simulink model "gyroPendulum"  (R2018a)
settings: Solver=FixedStepDiscrete  StartTime=0.0  StopTime=inf  FixedStep=timeStep  RelTol=1e-3
values from neighbouring files (symbols this model uses):
  alphaCoefficientsTable = [0.135955504695 0.137071048508 0.137987859192 0.138554072268 0.138582246682 0.137829429264 0.135972150233 0.132577620353 0.127076345916 0.118749819988 0.106761570128 0.0902777777548 ... (122412 elements, 10201x12)]    [cachedAlphaCoefficientsTable.mat]    (also in setup.m = [alphaCoefficientsTable; K1(1, :), K1(2, :)])
  alphaCompareTable = [-171.7 -171.7 -171.7 -171.7 -171.7 -171.7 -171.7 -171.7 -171.7 -171.7 -171.7 -171.7 ... (51005 elements, 10201x5)]    [cachedAlphaCompareTable.mat]    (also in setup.m = [alphaCompareTable; index1 - alphaRegion, index1 + alphaRegi)
  coefficientsTensor = zeros(nLinearizations / nWorkers, nLinearizations, nLinearizations, nLinearizations, 12)    [alphaParallel.m]    (also in coefficientsTensor.mat = [0.0662688248156 0.0648277946669 0.0634135109587 0.062021453)
  K1 = [K1(1, :) K1(2, :)]    [alphaParallel.m]    (also in setup.m = lqr(Aw1, Bw1, diag([1, 1, 3, 1, 1, 1]), diag([6, 6])))
  K2 = lqr(Aw2, Bw2, diag([15, 1, 1, 5]), diag([15]))    [setup.m]
  K3 = lqr(Aw3, Bw3, diag([1, 1, 1, 1]), diag([1]))    [setup.m]
  modelParameters = rmfield(modelParameters, 'alph2')    [alphaParallel.m]    (also in setup.m)
  nLinearizations = 8    [alphaParallel.m]    (also in nLinearizations.mat = 32; setup.m = 100)
  shiftedVariables = [shiftedVariables; wholeVariables(:, 1) + abs(min(wholeVariables(:, 1), [], 2))]    [alphaParallel.m]    (also in shiftedVariables.mat = [0 0 0 0])
  trajectory = [0.204039137261 -0.389047482528 0.184950739835 -0.34807965922 0.208093560422 -0.397377880713 0.182464301801 -0.343183800683 0.212362955443 -0.406162696705 0.180157605825 -0.338633761035 ... (832 elements, 4x208)]    [trajectory.mat]
  trajectoryTimeStep = 0.005    [setup.m]
  trajectoryToWalk = [0.20348839193 -0.387921068139 0.185314050902 -0.348794213842 0.206937106898 -0.395034683488 0.18313781068 -0.34450971149 0.210555704125 -0.402555806913 0.181086396317 -0.340463307968 ... (484 elements, 4x121)]    [trajectoryToWalk.mat]
  trajectoryWalk = [0.250192072849 -0.608547594051 0.394694165643 -0.613804432575 0.251033796696 -0.60716129389 0.397031433715 -0.614641196656 0.251771384595 -0.605603254171 0.399919372114 -0.616088285913 ... (1104 elements, 4x276)]    [trajectoryWalk.mat]
  variablesDeltas = [variablesDeltas; abs(variablesRanges(2:end, 1) - variablesRanges(2:end, 2)) / nLinearizations]    [alphaParallel.m]    (also in variablesDeltas.mat = [16.875 5.625 5.625 5.625])
  variablesShift = [variablesShift; abs(min(wholeVariables, [], 2))]    [alphaParallel.m]    (also in variablesShift.mat = [270 90 90 90])
undefined symbols (not defined in the file or in its folder): DiscIntNeverNeededParam
libraries: simulink x15, dspindex x12, simulink_extras x5
settings Model: EnablePacing=on  PacingRate=2  Creator=Oleg  LastModifiedBy=sorok

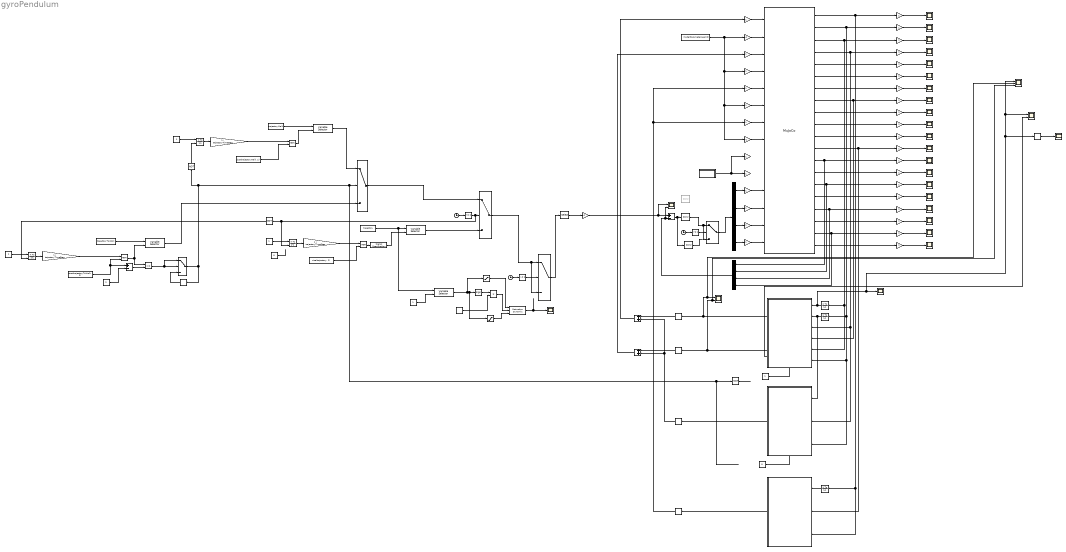
== system gyroPendulum ==
  Add : Sum
  Add1 : Sum
  Clock : Clock
  Clock1 : Clock
  Clock2 : Clock
  Compare To Constant : simulink/Logic and Bit Operations/Compare To Constant  relop=>=  const=2  OutDataTypeStr=boolean
  Compare To Constant1 : simulink/Logic and Bit Operations/Compare To Constant  relop=>=  const=2  OutDataTypeStr=boolean
  Compare To Constant2 : simulink/Logic and Bit Operations/Compare To Constant  relop=>=  const=1  OutDataTypeStr=boolean
  Constant : Constant  Value=modelParameters.gamD
  Constant1 : Constant  Value=size(trajectory, 2)
  Constant10 : Constant  Value=2
  Constant11 : Constant
  Constant12 : Constant  Value=0
  Constant13 : Constant  Value=0
  Constant14 : Constant
  Constant2 : Constant  SampleTime=trajectoryTimeStep
  Constant3 : Constant  Value=trajectory
  Constant4 : Constant  Value=size(trajectoryWalk, 2)
  Constant5 : Constant  SampleTime=trajectoryTimeStep
  Constant6 : Constant  Value=trajectoryWalk
  Constant7 : Constant  Value=size(trajectoryToWalk, 2)
  Constant8 : Constant  SampleTime=trajectoryTimeStep
  Constant9 : Constant  Value=trajectoryToWalk
  Demux : Demux
  Discrete-Time Integrator : DiscreteIntegrator  ExternalReset=level  SampleTime=-1  ICPrevOutput=DiscIntNeverNeededParam  ICPrevScaledInput=DiscIntNeverNeededParam
  Discrete-Time Integrator1 : DiscreteIntegrator  SampleTime=-1  ICPrevOutput=DiscIntNeverNeededParam  ICPrevScaledInput=DiscIntNeverNeededParam
  Discrete-Time Integrator2 : DiscreteIntegrator  SampleTime=-1  ICPrevOutput=DiscIntNeverNeededParam  ICPrevScaledInput=DiscIntNeverNeededParam
  Discrete-Time Integrator3 : DiscreteIntegrator  SampleTime=-1  ICPrevOutput=DiscIntNeverNeededParam  ICPrevScaledInput=DiscIntNeverNeededParam
  Discrete-Time Integrator4 : DiscreteIntegrator  ExternalReset=level  SampleTime=-1  ICPrevOutput=DiscIntNeverNeededParam  ICPrevScaledInput=DiscIntNeverNeededParam
  Discrete-Time Integrator5 : DiscreteIntegrator  ExternalReset=level  SampleTime=-1  ICPrevOutput=DiscIntNeverNeededParam  ICPrevScaledInput=DiscIntNeverNeededParam
  Disturbances : Subsystem
  Equal : RelationalOperator  OutDataTypeStr=boolean  RndMeth=Simplest
  Gain : Gain  Gain=1 / trajectoryTimeStep
  Gain1 : Gain  Gain=1 / trajectoryTimeStep
  Gain2 : Gain  Gain=1 / trajectoryTimeStep
  Gain3 : Gain  Gain=-1
  Memory{,1..4} (5 alike) : Memory
  Minus : Sum  Inputs=+-
  Minus1 : Sum  Inputs=+-
  Multiply : Product
  Mux1 : Mux
  NOT : Logic  Operator=NOT  IconShape=distinctive  AllPortsSameDT=off  OutDataTypeStr=boolean
  NOT1 : Logic  Operator=NOT  IconShape=distinctive  AllPortsSameDT=off  OutDataTypeStr=boolean
  NOT2 : Logic  Operator=NOT  IconShape=distinctive  AllPortsSameDT=off  OutDataTypeStr=boolean
  PID Controller : simulink/Continuous/PID Controller  Controller=PD  TimeDomain=Discrete-time  SampleTime=-1  IntegratorMethod=Forward Euler  FilterMethod=Forward Euler  Form=Parallel  UseFilter=on  ControllerParametersSource=internal  P=350  I=1  D=350  N=100  InitialConditionSource=internal  InitialConditionForIntegrator=0  InitialConditionForFilter=0  ExternalReset=none  LimitOutput=off  UpperSaturationLimit=inf  LowerSaturationLimit=-inf  LinearizeAsGain=on  AntiWindupMode=none  Kb=1  TrackingMode=off  Kt=1  PParamMin=[]  PParamMax=[]  IParamMin=[]  IParamMax=[]  DParamMin=[]  DParamMax=[]  NParamMin=[]  NParamMax=[]  KbParamMin=[]  KbParamMax=[]  KtParamMin=[]  KtParamMax=[]  POutMin=[]  POutMax=[]  IOutMin=[]  IOutMax=[]  DOutMin=[]  DOutMax=[]  NOutMin=[]  NOutMax=[]  KbOutMin=[]  KbOutMax=[]  KtOutMin=[]  KtOutMax=[]  IntegratorOutMin=[]  IntegratorOutMax=[]  FilterOutMin=[]  FilterOutMax=[]  SumOutMin=[]  SumOutMax=[]  SumI1OutMin=[]  SumI1OutMax=[]  SumI2OutMin=[]  SumI2OutMax=[]  SumI3OutMin=[]  SumI3OutMax=[]  SumDOutMin=[]  SumDOutMax=[]  SaturationOutMin=[]  SaturationOutMax=[]  IntegratorContinuousStateAttributes=''  IntegratorStateMustResolveToSignalObject=off  IntegratorRTWStateStorageClass=Auto  FilterContinuousStateAttributes=''  FilterStateMustResolveToSignalObject=off  FilterRTWStateStorageClass=Auto  DifferentiatorICPrevScaledInput=0  DifferentiatorOutMin=[]  DifferentiatorOutMax=[]  FilterDiffOutCoefMin=[]  FilterDiffOutCoefMax=[]  SumDenOutMin=[]  SumDenOutMax=[]  SumNumOutMin=[]  SumNumOutMax=[]  ReciprocalOutMin=[]  ReciprocalOutMax=[]  DivideOutMin=[]  DivideOutMax=[]  TunerSelectOption=Transfer Function Based (PID Tuner App)
  PID Controller1 : simulink/Continuous/PID Controller  Commented=on  Controller=PD  TimeDomain=Discrete-time  SampleTime=-1  IntegratorMethod=Forward Euler  FilterMethod=Forward Euler  Form=Parallel  UseFilter=on  ControllerParametersSource=internal  P=300  I=1  D=300  N=100  InitialConditionSource=internal  InitialConditionForIntegrator=0  InitialConditionForFilter=0  ExternalReset=none  LimitOutput=off  UpperSaturationLimit=inf  LowerSaturationLimit=-inf  LinearizeAsGain=on  AntiWindupMode=none  Kb=1  TrackingMode=off  Kt=1  PParamMin=[]  PParamMax=[]  IParamMin=[]  IParamMax=[]  DParamMin=[]  DParamMax=[]  NParamMin=[]  NParamMax=[]  KbParamMin=[]  KbParamMax=[]  KtParamMin=[]  KtParamMax=[]  POutMin=[]  POutMax=[]  IOutMin=[]  IOutMax=[]  DOutMin=[]  DOutMax=[]  NOutMin=[]  NOutMax=[]  KbOutMin=[]  KbOutMax=[]  KtOutMin=[]  KtOutMax=[]  IntegratorOutMin=[]  IntegratorOutMax=[]  FilterOutMin=[]  FilterOutMax=[]  SumOutMin=[]  SumOutMax=[]  SumI1OutMin=[]  SumI1OutMax=[]  SumI2OutMin=[]  SumI2OutMax=[]  SumI3OutMin=[]  SumI3OutMax=[]  SumDOutMin=[]  SumDOutMax=[]  SaturationOutMin=[]  SaturationOutMax=[]  IntegratorContinuousStateAttributes=''  IntegratorStateMustResolveToSignalObject=off  IntegratorRTWStateStorageClass=Auto  FilterContinuousStateAttributes=''  FilterStateMustResolveToSignalObject=off  FilterRTWStateStorageClass=Auto  DifferentiatorICPrevScaledInput=0  DifferentiatorOutMin=[]  DifferentiatorOutMax=[]  FilterDiffOutCoefMin=[]  FilterDiffOutCoefMax=[]  SumDenOutMin=[]  SumDenOutMax=[]  SumNumOutMin=[]  SumNumOutMax=[]  ReciprocalOutMin=[]  ReciprocalOutMax=[]  DivideOutMin=[]  DivideOutMax=[]  TunerSelectOption=Transfer Function Based (PID Tuner App)
  PID Controller2 : simulink/Continuous/PID Controller  Controller=PD  TimeDomain=Discrete-time  SampleTime=-1  IntegratorMethod=Forward Euler  FilterMethod=Forward Euler  Form=Parallel  UseFilter=on  ControllerParametersSource=internal  P=200  I=1  D=200  N=100  InitialConditionSource=internal  InitialConditionForIntegrator=0  InitialConditionForFilter=0  ExternalReset=none  LimitOutput=off  UpperSaturationLimit=inf  LowerSaturationLimit=-inf  LinearizeAsGain=on  AntiWindupMode=none  Kb=1  TrackingMode=off  Kt=1  PParamMin=[]  PParamMax=[]  IParamMin=[]  IParamMax=[]  DParamMin=[]  DParamMax=[]  NParamMin=[]  NParamMax=[]  KbParamMin=[]  KbParamMax=[]  KtParamMin=[]  KtParamMax=[]  POutMin=[]  POutMax=[]  IOutMin=[]  IOutMax=[]  DOutMin=[]  DOutMax=[]  NOutMin=[]  NOutMax=[]  KbOutMin=[]  KbOutMax=[]  KtOutMin=[]  KtOutMax=[]  IntegratorOutMin=[]  IntegratorOutMax=[]  FilterOutMin=[]  FilterOutMax=[]  SumOutMin=[]  SumOutMax=[]  SumI1OutMin=[]  SumI1OutMax=[]  SumI2OutMin=[]  SumI2OutMax=[]  SumI3OutMin=[]  SumI3OutMax=[]  SumDOutMin=[]  SumDOutMax=[]  SaturationOutMin=[]  SaturationOutMax=[]  IntegratorContinuousStateAttributes=''  IntegratorStateMustResolveToSignalObject=off  IntegratorRTWStateStorageClass=Auto  FilterContinuousStateAttributes=''  FilterStateMustResolveToSignalObject=off  FilterRTWStateStorageClass=Auto  DifferentiatorICPrevScaledInput=0  DifferentiatorOutMin=[]  DifferentiatorOutMax=[]  FilterDiffOutCoefMin=[]  FilterDiffOutCoefMax=[]  SumDenOutMin=[]  SumDenOutMax=[]  SumNumOutMin=[]  SumNumOutMax=[]  ReciprocalOutMin=[]  ReciprocalOutMax=[]  DivideOutMin=[]  DivideOutMax=[]  TunerSelectOption=Transfer Function Based (PID Tuner App)
  Pitch controller (3 dimensions) : Subsystem
  Pitch-yaw controller (7 dimensions) : Subsystem
  Radians to Degrees : simulink_extras/Transformations/Radians to Degrees
  Ramp : simulink/Sources/Ramp  slope=0.2  start=0  InitialOutput=0
  Rem : Math  Operator=rem  SaturateOnIntegerOverflow=on
  Rem1 : Math  Operator=rem  SaturateOnIntegerOverflow=on
  Rem2 : Math  Operator=rem  SaturateOnIntegerOverflow=on
  Roll controller (3 dimensions) : Subsystem
  S-Function : S-Function  FunctionName=MuJoCo  SFunctionDeploymentMode=off  EnableBusSupport=off
  Saturation : Saturate  UpperLimit=inf  LowerLimit=0
  Saturation Dynamic : simulink/Discontinuities/Saturation Dynamic  OutMin=[]  OutMax=[]  OutDataTypeStr=Inherit: Same as second input  OutDataType=fixdt(1, 16)  OutScaling=2^-10  DoSatur=off
  Saturation1 : Saturate  UpperLimit=0  LowerLimit=-inf
  Scope{,1..5,7..21,24,26} (23 alike) : Scope
  Scope22 : Scope  NumInputPorts=3
  Scope23 : Scope  NumInputPorts=2
  Scope25 : Scope  NumInputPorts=2
  Scope6 : Scope  NumInputPorts=2
  Selector1 : Selector  InputPortWidth=4  IndexOptions=Index vector (dialog)  Indices=[3 4 1 2]  OutputSizes=1
  Sign : Signum
  Signal Specification : SignalSpecification  Dimensions=1
  Switch{,1..4} (5 alike) : Switch  Criteria=u2 > Threshold
  Variable Selector{,1..3} (4 alike) : dspindex/Variable Selector  NumInputs=1  rowsOrCols=Columns  IdxMode=Variable  Elements=[1 3]  ZerOneIdxMode=One-based  errmode=Clip Index  FillMode=on  FillValues=0
  gyro1_act : Gain
  gyro1_act_pos : Gain
  gyro1_act_vel : Gain
  gyro1_m : Gain  Gain=-1
  gyro1_m_pos : Gain
  gyro1_m_vel : Gain
  gyro2_act : Gain
  gyro2_act_pos : Gain
  gyro2_act_vel : Gain
  gyro2_m : Gain
  gyro2_m_pos : Gain
  gyro2_m_vel : Gain
  gyro3_act : Gain
  gyro3_act_pos : Gain
  gyro3_m : Gain
  gyro4_act : Gain
  gyro4_m : Gain  Gain=-1
  ls_act : Gain
  ls_pos : Gain
  ls_vel : Gain
  lt_act : Gain
  lt_pos : Gain
  lt_vel : Gain
  rod_act1 : Gain
  rod_act2 : Gain
  rod_x_ang : Gain
  rod_y_ang : Gain
  rod_z_ang : Gain
  rs_act : Gain
  rs_pos : Gain
  rs_vel : Gain
  rt_act : Gain
  rt_pos : Gain
  rt_vel : Gain
  wires:
  rod_x_ang/1 -> Scope/1
  gyro1_act_pos/1 -> Scope2/1
  rod_y_ang/1 -> Scope1/1
  gyro1_act_vel/1 -> Scope3/1
  gyro1_m_pos/1 -> Scope4/1
  gyro1_m_vel/1 -> Scope5/1
  Constant/1 -> gyro4_m/1, gyro3_m/1, gyro2_m/1, gyro1_m/1
  Pitch-yaw controller (7 dimensions)/1(alph1D) -> Scope22/2, Scope6/1, Memory1/1
  Memory1/1 -> Add/1
  gyro1_m/1 -> S-Function/2
  gyro2_act/1 -> S-Function/3
  gyro2_m/1 -> S-Function/4
  gyro2_m_vel/1 -> Scope11/1
  gyro2_m_pos/1 -> Scope10/1
  gyro2_act_vel/1 -> Scope9/1
  gyro2_act_pos/1 -> Scope8/1
  rod_z_ang/1 -> Scope12/1
  Pitch-yaw controller (7 dimensions)/2(alph2D) -> Scope22/3, Scope6/2, Memory2/1
  gyro1_act/1 -> S-Function/1
  Memory2/1 -> Add1/1
  Disturbances/1(Out) -> rod_act1/1, rod_act2/1
  Constant3/1 -> Variable Selector3/1, Variable Selector/1
  Variable Selector/1 -> Switch/3
  Discrete-Time Integrator/1 -> Gain/1
  Constant1/1 -> Rem/2
  Rem/1 -> Signal Specification/1
  Clock/1 -> Compare To Constant/1
  gyro3_m/1 -> S-Function/6
  gyro4_m/1 -> S-Function/8
  gyro3_act/1 -> S-Function/5
  gyro4_act/1 -> S-Function/7
  gyro3_act_pos/1 -> Scope7/1
  Memory3/1 -> gyro3_act/1, gyro4_act/1
  Compare To Constant/1 -> Discrete-Time Integrator/2, NOT/1, Switch/2
  Constant2/1 -> Discrete-Time Integrator/1
  Switch/1 -> Switch3/3, Switch3/1
  S-Function/1 -> Discrete-Time Integrator3/1, Roll controller (3 dimensions)/3(sigmD), rod_x_ang/1
  S-Function/2 -> Discrete-Time Integrator2/1, Pitch controller (3 dimensions)/3(thetD), Pitch-yaw controller (7 dimensions)/6(thetD), rod_y_ang/1
  S-Function/3 -> Discrete-Time Integrator1/1, Pitch-yaw controller (7 dimensions)/5(psihD), rod_z_ang/1
  S-Function/4 -> Pitch-yaw controller (7 dimensions)/3(alph1), Pitch controller (3 dimensions)/2(alph1), gyro1_act_pos/1
  S-Function/5 -> gyro1_act_vel/1
  S-Function/6 -> gyro1_m_pos/1
  S-Function/7 -> gyro1_m_vel/1
  S-Function/8 -> Pitch-yaw controller (7 dimensions)/4(alph2), gyro2_act_pos/1
  S-Function/9 -> gyro2_act_vel/1
  S-Function/10 -> gyro2_m_pos/1
  S-Function/11 -> gyro2_m_vel/1
  S-Function/12 -> gyro3_act_pos/1, Roll controller (3 dimensions)/2(alph3)
  Gain/1 -> Rem/1
  Discrete-Time Integrator1/1 -> Pitch-yaw controller (7 dimensions)/1(psih), Radians to Degrees/1, Scope23/1, Scope22/1, Scope21/1
  Discrete-Time Integrator2/1 -> Pitch-yaw controller (7 dimensions)/2(thet), Pitch controller (3 dimensions)/1(thet)
  Discrete-Time Integrator3/1 -> Roll controller (3 dimensions)/1(sigm)
  S-Function/14 -> lt_vel/1
  S-Function/13 -> Mux1/1, lt_pos/1
  S-Function/15 -> Mux1/2, ls_pos/1
  S-Function/16 -> ls_vel/1
  S-Function/17 -> Mux1/3, rt_pos/1
  S-Function/18 -> rt_vel/1
  S-Function/19 -> Mux1/4, rs_pos/1
  S-Function/20 -> rs_vel/1
  lt_pos/1 -> Scope13/1
  lt_vel/1 -> Scope14/1
  ls_pos/1 -> Scope15/1
  ls_vel/1 -> Scope16/1
  rt_pos/1 -> Scope17/1
  rt_vel/1 -> Scope18/1
  rs_pos/1 -> Scope19/1
  rs_vel/1 -> Scope20/1
  Demux/1 -> lt_act/1
  Demux/2 -> ls_act/1
  Demux/3 -> rt_act/1
  Demux/4 -> rs_act/1
  Minus/1 -> PID Controller2/1, PID Controller/1
  Mux1/1 -> Scope25/2, Minus/2
  Gain1/1 -> Rem1/1
  Constant5/1 -> Discrete-Time Integrator4/1
  Rem1/1 -> Variable Selector1/2
  Constant4/1 -> Rem1/2
  Discrete-Time Integrator4/1 -> Gain1/1
  Variable Selector1/1 -> Switch1/1
  Constant6/1 -> Variable Selector1/1
  NOT/1 -> Discrete-Time Integrator5/2
  Discrete-Time Integrator5/1 -> Gain2/1
  Constant8/1 -> Discrete-Time Integrator5/1
  Constant9/1 -> Variable Selector2/1
  Constant7/1 -> Minus1/1, Rem2/2
  Gain2/1 -> Rem2/1
  Rem2/1 -> Equal/1, Variable Selector2/2
  Equal/1 -> Switch2/1, Switch2/2
  Switch2/1 -> NOT1/1, Switch1/2, NOT2/1, Memory/1
  Memory/1 -> Switch2/3
  Switch1/1 -> Switch/1
  Variable Selector2/1 -> Switch1/3
  NOT1/1 -> Discrete-Time Integrator4/2
  Minus1/1 -> Equal/2
  Constant10/1 -> Minus1/2
  NOT2/1 -> ?
  Pitch controller (3 dimensions)/1(alph1D) -> Memory4/1
  Memory4/1 -> Add/2, Add1/2
  Add/1 -> gyro1_act/1
  Add1/1 -> gyro2_act/1
  Constant11/1 -> Pitch-yaw controller (7 dimensions)/Enable
  Constant12/1 -> Pitch controller (3 dimensions)/Enable
  Selector1/1 -> Gain3/1
  Roll controller (3 dimensions)/1(alph3D) -> Memory3/1
  PID Controller/1 -> Switch4/3, Switch4/1
  Gain3/1 -> Scope25/1, Minus/1
  Pitch-yaw controller (7 dimensions)/3(Output) -> Scope23/2
  Clock1/1 -> Compare To Constant1/1
  Compare To Constant1/1 -> Switch3/2
  Constant14/1 -> Variable Selector3/2
  Variable Selector3/1 -> Saturation/1, Saturation1/1, Sign/1
  Switch3/1 -> Selector1/1
  Compare To Constant2/1 -> Switch4/2
  Clock2/1 -> Compare To Constant2/1
  Switch4/1 -> Demux/1
  PID Controller2/1 -> ?
  Ramp/1 -> Multiply/2
  Saturation Dynamic/1 -> Scope24/1
  Sign/1 -> Multiply/1
  Multiply/1 -> Saturation Dynamic/2
  Saturation/1 -> Saturation Dynamic/1
  Saturation1/1 -> Saturation Dynamic/3
  Constant13/1 -> ?
  Signal Specification/1 -> Variable Selector/2
  lt_act/1 -> S-Function/11
  ls_act/1 -> S-Function/12
  rt_act/1 -> S-Function/13
  rs_act/1 -> S-Function/14
  Radians to Degrees/1 -> Scope26/1

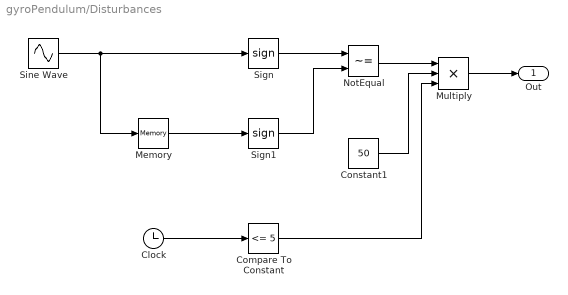
== system gyroPendulum/Disturbances ==
  Clock : Clock
  Compare To Constant : simulink/Logic and Bit Operations/Compare To Constant  relop=<=  const=5  OutDataTypeStr=boolean
  Constant1 : Constant  Value=50
  Memory : Memory
  Multiply : Product  Inputs=3
  NotEqual : RelationalOperator  Operator=~=  OutDataTypeStr=boolean  RndMeth=Simplest
  Sign : Signum
  Sign1 : Signum
  Sine Wave : Sin  Frequency=2  Phase=-0.5  SampleTime=0
  Out : Outport
  wires:
  Constant1/1 -> Multiply/2
  Multiply/1 -> Out/1
  Sign/1 -> NotEqual/1
  Sine Wave/1 -> Memory/1, Sign/1
  Clock/1 -> Compare To Constant/1
  NotEqual/1 -> Multiply/1
  Compare To Constant/1 -> Multiply/3
  Memory/1 -> Sign1/1
  Sign1/1 -> NotEqual/2

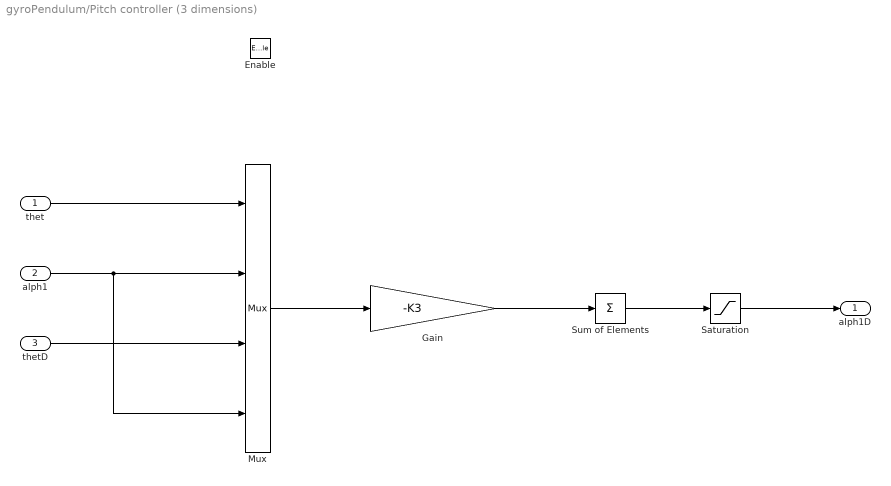
== system gyroPendulum/Pitch controller (3 dimensions) ==
  thet : Inport
  alph1 : Inport  Port=2
  thetD : Inport  Port=3
  Enable : EnablePort  StatesWhenEnabling=reset
  Gain : Gain  Gain=-K3
  Mux : Mux
  Saturation : Saturate  UpperLimit=3  LowerLimit=-3
  Sum of Elements : Sum  Inputs=+
  alph1D : Outport
  wires:
  thetD/1 -> Mux/3
  thet/1 -> Mux/1
  Mux/1 -> Gain/1
  Gain/1 -> Sum of Elements/1
  Sum of Elements/1 -> Saturation/1
  Saturation/1 -> alph1D/1
  alph1/1 -> Mux/4, Mux/2

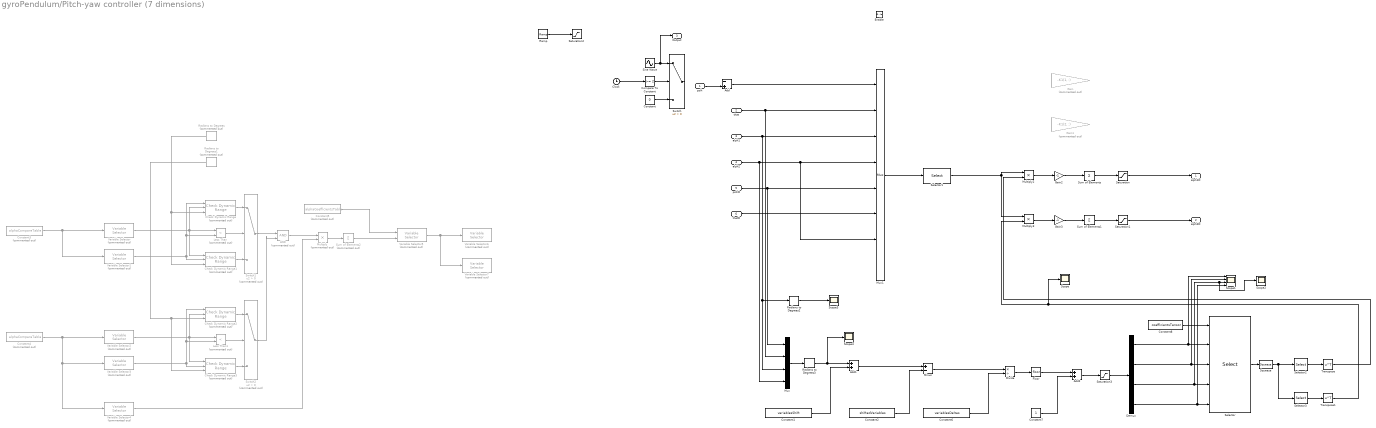
== system gyroPendulum/Pitch-yaw controller (7 dimensions) ==
  psih : Inport
  thet : Inport  Port=2
  alph1 : Inport  Port=3
  alph2 : Inport  Port=4
  psihD : Inport  Port=5
  thetD : Inport  Port=6
  Enable : EnablePort  StatesWhenEnabling=reset
  AND : Logic  Commented=on  IconShape=distinctive  AllPortsSameDT=off  OutDataTypeStr=boolean
  Add : Sum  Inputs=-+
  Add1 : Sum
  Add2 : Sum
  Check Dynamic Range{,1..3} (4 alike) : simulink/Model Verification/Check  Dynamic Range  Description=min < u < max  Commented=on  enabled=off  stopWhenAssertionFail=off  export=on  icon=graphic
      settings: SourceProductName=Simulink  SourceProductBaseCode=SL
  Clock : Clock
  Compare To Constant : simulink/Logic and Bit Operations/Compare To Constant  relop=>=  const=2  OutDataTypeStr=boolean
  Constant : Constant  Value=0
  Constant1 : Constant  Value=variablesShift
  Constant2 : Constant  Value=shiftedVariables
  Constant3 : Constant  Commented=on  Value=alphaCompareTable
  Constant4 : Constant  Commented=on  Value=alphaCompareTable
  Constant5 : Constant  Commented=on  Value=alphaCoefficientsTable
  Constant6 : Constant  Value=variablesDeltas
  Constant7 : Constant
  Constant8 : Constant  Value=coefficientsTensor
  Demux : Demux
  Divide : Product  Inputs=*/
  Floor : Rounding
  Gain : Gain  Commented=on  Gain=-K1(1, :)
  Gain1 : Gain  Commented=on  Gain=-K1(2, :)
  Gain2 : Gain  Gain=-1
  Gain3 : Gain  Gain=-1
  Less Than : RelationalOperator  Commented=on  Operator=<  OutDataTypeStr=boolean  RndMeth=Simplest
  Less Than1 : RelationalOperator  Commented=on  Operator=<  OutDataTypeStr=boolean  RndMeth=Simplest
  Minus : Sum  Inputs=+-
  Multiply : Product  Commented=on
  Multiply2 : Product
  Multiply3 : Product
  Mux : Mux
  Mux1 : Mux  Inputs=8
  Radians to Degrees : simulink_extras/Transformations/Radians to Degrees  Commented=on
  Radians to Degrees1 : simulink_extras/Transformations/Radians to Degrees  Commented=on
  Radians to Degrees2 : simulink_extras/Transformations/Radians to Degrees
  Radians to Degrees3 : simulink_extras/Transformations/Radians to Degrees
  Ramp : simulink/Sources/Ramp  slope=0.09  start=0  InitialOutput=0
  Saturation : Saturate  UpperLimit=4.5  LowerLimit=-4.5
  Saturation1 : Saturate  UpperLimit=4.5  LowerLimit=-4.5
  Saturation2 : Saturate  UpperLimit=45 / 180 * pi  LowerLimit=0
  Saturation3 : Saturate  UpperLimit=nLinearizations  LowerLimit=1
  Scope{,2..4} (4 alike) : Scope
  Scope1 : Scope  NumInputPorts=4
  Selector : Selector  NumberOfDimensions=5  InputPortWidth=3  IndexOptions=Index vector (port),Index vector (port),Index vector (port),Index vector (port),Select all  Indices=[1 3],1,1,1,1  OutputSizes=1,1,1,1,1
  Selector1 : Selector  NumberOfDimensions=2  InputPortWidth=7  IndexOptions=Index vector (dialog),Index vector (dialog)  Indices=1,[1 2 4 5 6 7]  OutputSizes=1,1
  Selector2 : Selector  InputPortWidth=12  IndexOptions=Index vector (dialog)  Indices=1:6  OutputSizes=1
  Selector3 : Selector  InputPortWidth=12  IndexOptions=Index vector (dialog)  Indices=7:12  OutputSizes=1
  Sine Wave : Sin  Amplitude=45 / 180 * pi  Frequency=0.75  SampleTime=0
  Squeeze : Squeeze
  Sum of Elements : Sum  Inputs=+
  Sum of Elements1 : Sum  Inputs=+
  Sum of Elements2 : Sum  Commented=on  Inputs=+
  Switch : Switch  Criteria=u2 > Threshold
  Switch1 : Switch  Commented=on  Criteria=u2 > Threshold
  Switch2 : Switch  Commented=on  Criteria=u2 > Threshold
  Transpose : Math  Operator=transpose  SaturateOnIntegerOverflow=on
  Transpose1 : Math  Operator=transpose  SaturateOnIntegerOverflow=on
  Variable Selector : dspindex/Variable Selector  Commented=on  NumInputs=1  rowsOrCols=Columns  IdxMode=Fixed  Elements=1  ZerOneIdxMode=One-based  errmode=Clip Index  FillMode=on  FillValues=0
  Variable Selector1 : dspindex/Variable Selector  Commented=on  NumInputs=1  rowsOrCols=Columns  IdxMode=Fixed  Elements=2  ZerOneIdxMode=One-based  errmode=Clip Index  FillMode=on  FillValues=0
  Variable Selector2 : dspindex/Variable Selector  Commented=on  NumInputs=1  rowsOrCols=Columns  IdxMode=Fixed  Elements=3  ZerOneIdxMode=One-based  errmode=Clip Index  FillMode=on  FillValues=0
  Variable Selector3 : dspindex/Variable Selector  Commented=on  NumInputs=1  rowsOrCols=Columns  IdxMode=Fixed  Elements=4  ZerOneIdxMode=One-based  errmode=Clip Index  FillMode=on  FillValues=0
  Variable Selector4 : dspindex/Variable Selector  Commented=on  NumInputs=1  rowsOrCols=Columns  IdxMode=Fixed  Elements=5  ZerOneIdxMode=One-based  errmode=Clip Index  FillMode=on  FillValues=0
  Variable Selector5 : dspindex/Variable Selector  Commented=on  NumInputs=1  rowsOrCols=Rows  IdxMode=Variable  Elements=[1 3]  ZerOneIdxMode=One-based  errmode=Clip Index  FillMode=on  FillValues=0
  Variable Selector6 : dspindex/Variable Selector  Commented=on  NumInputs=1  rowsOrCols=Columns  IdxMode=Fixed  Elements=1:6  ZerOneIdxMode=One-based  errmode=Clip Index  FillMode=on  FillValues=0
  Variable Selector7 : dspindex/Variable Selector  Commented=on  NumInputs=1  rowsOrCols=Columns  IdxMode=Fixed  Elements=7:12  ZerOneIdxMode=One-based  errmode=Clip Index  FillMode=on  FillValues=0
  alph1D : Outport
  alph2D : Outport  Port=2
  Output : Outport  Port=3
  wires:
  Multiply2/1 -> Gain2/1
  Sum of Elements/1 -> Saturation/1
  Saturation/1 -> alph1D/1
  Multiply3/1 -> Gain3/1
  Sum of Elements1/1 -> Saturation1/1
  Saturation1/1 -> alph2D/1
  Clock/1 -> Compare To Constant/1
  Compare To Constant/1 -> Switch/2
  Add/1 -> Mux1/1
  Constant/1 -> Switch/3
  psih/1 -> Add/2
  thet/1 -> Mux/2, Mux1/2
  psihD/1 -> Mux/1, Mux1/5
  thetD/1 -> Mux1/6
  Mux1/1 -> Selector1/1
  Selector1/1 -> Multiply3/1, Multiply2/1
  Ramp/1 -> Saturation2/1
  Sine Wave/1 -> Switch/1, Output/1
  alph1/1 -> Radians to Degrees2/1, Mux/3, Mux1/3
  alph2/1 -> Mux/4, Mux1/7, Mux1/4
  AND/1 -> Multiply/1
  Switch2/1 -> AND/2
  Constant5/1 -> Variable Selector5/1
  Variable Selector3/1 -> Check Dynamic Range3/2, Less Than1/2, Check Dynamic Range2/1
  Multiply/1 -> Sum of Elements2/1
  Switch1/1 -> AND/1
  Constant4/1 -> Variable Selector2/1, Variable Selector4/1, Variable Selector3/1
  Less Than1/1 -> Switch2/2
  Radians to Degrees1/1 -> Check Dynamic Range2/3, Check Dynamic Range3/3
  Check Dynamic Range3/1 -> Switch2/3
  Check Dynamic Range2/1 -> Switch2/1
  Check Dynamic Range1/1 -> Switch1/3
  Variable Selector/1 -> Check Dynamic Range/2, Check Dynamic Range1/1, Less Than/1
  Constant3/1 -> Variable Selector1/1, Variable Selector/1
  Variable Selector4/1 -> Multiply/2
  Less Than/1 -> Switch1/2
  Variable Selector2/1 -> Less Than1/1, Check Dynamic Range3/1, Check Dynamic Range2/2
  Radians to Degrees/1 -> Check Dynamic Range1/3, Check Dynamic Range/3
  Sum of Elements2/1 -> Variable Selector5/2
  Variable Selector1/1 -> Check Dynamic Range/1, Less Than/2, Check Dynamic Range1/2
  Check Dynamic Range/1 -> Switch1/1
  Variable Selector5/1 -> Variable Selector7/1, Variable Selector6/1
  Gain2/1 -> Sum of Elements/1
  Gain3/1 -> Sum of Elements1/1
  Mux/1 -> Radians to Degrees3/1
  Add1/1 -> Minus/1
  Minus/1 -> Divide/1
  Constant1/1 -> Add1/2
  Constant2/1 -> Minus/2
  Constant6/1 -> Divide/2
  Divide/1 -> Floor/1
  Floor/1 -> Add2/1
  Constant7/1 -> Add2/2
  Constant8/1 -> Selector/1
  Demux/2 -> Scope1/2, Selector/3
  Demux/3 -> Scope2/1, Scope1/3, Selector/4
  Demux/4 -> Scope1/4, Selector/5
  Add2/1 -> Saturation3/1
  Selector/1 -> Squeeze/1
  Selector2/1 -> Transpose/1
  Selector3/1 -> Transpose1/1
  Squeeze/1 -> Selector3/1, Selector2/1
  Transpose/1 -> Multiply2/2
  Transpose1/1 -> Scope/1, Multiply3/2
  Demux/1 -> Scope1/1, Selector/2
  Radians to Degrees2/1 -> Scope3/1
  Radians to Degrees3/1 -> Scope4/1, Add1/1
  Saturation3/1 -> Demux/1

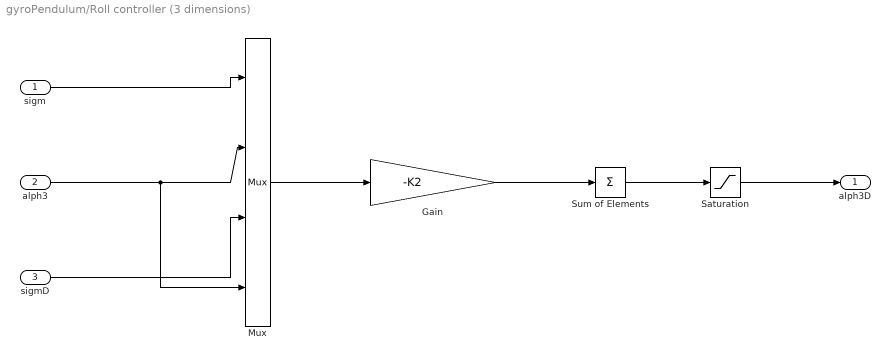
== system gyroPendulum/Roll controller (3 dimensions) ==
  sigm : Inport
  alph3 : Inport  Port=2
  sigmD : Inport  Port=3
  Gain : Gain  Gain=-K2
  Mux : Mux
  Saturation : Saturate  UpperLimit=3  LowerLimit=-3
  Sum of Elements : Sum  Inputs=+
  alph3D : Outport
  wires:
  Saturation/1 -> alph3D/1
  Sum of Elements/1 -> Saturation/1
  Gain/1 -> Sum of Elements/1
  Mux/1 -> Gain/1
  alph3/1 -> Mux/4, Mux/2
  sigm/1 -> Mux/1
  sigmD/1 -> Mux/3
